simulink model "Copy_of_PDUSTM32"  (R2024b)
settings: Solver=FixedStepDiscrete  StartTime=0.0  StopTime=1  FixedStep=0.001  RelTol=1e-3  EnableMultiTasking=on
libraries: stm32blockslib x32, stm32f4xxblockslib x14, canmsglib x7, simulink x3, stm32h7xxblockslib x1
(part 2 of 3)

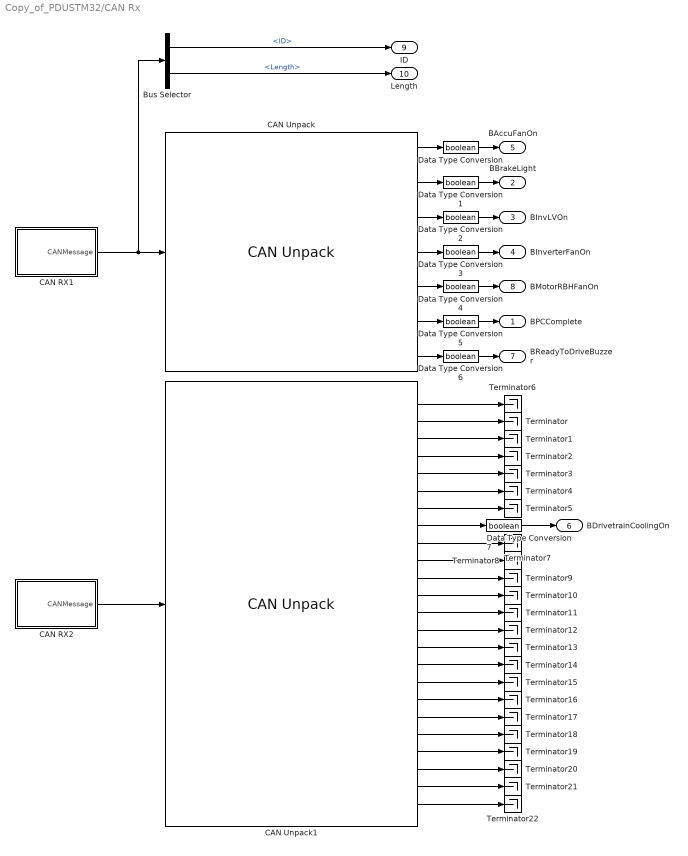
== system Copy_of_PDUSTM32/CAN Rx ==
  Bus Selector : BusSelector  OutputSignals=ID,Length
  CAN RX1 : Subsystem  mask{SPIModuleSelect=SPI1, Port_Select=GPIOB, Pin=14, PortName=GPIOB, PinNumber=2}
      mask prompts: SPIModuleSelect "SPI Module"; Port_Select "CS Port"; Pin "CS Pin"; PortName "INT Port"; PinNumber "INT Pin"
      mask TypeOptions SPIModuleSelect:
      | Enabled
      | Subsystem/SPI Controller Transfer7/SPIModuleSelect
      mask TypeOptions Port_Select:
      | Enabled
      | Subsystem/SPI Controller Transfer7/Port_Select
      mask TypeOptions Pin:
      | Enabled
      | Subsystem/SPI Controller Transfer7/Pin
      mask TypeOptions PortName: Digital Port Read5/PortName
      mask TypeOptions PinNumber: Digital Port Read5/PinNumber
      mask DialogControl DescTextVar Prompt: Read RX buffer when the INT pin is pulled low. Outputs a CANMessage type to be fed into a CAN unpack
      mask Display:
      | %port_label('output', 1, 'CANMessage');
      | 
      | text(0.05, 0.5, '' + string(get_param(gcb,'SPIModuleSelect')), HorizontalAlignment = 'left');
      | text(0.05, 0.85, 'CS ' + string(get_param(gcb,'Port_Select')) + ' Pin ' + string(get_param(gcb,'Pin')), HorizontalAlignment = 'left');
      | 
      | 
      | text(0.05, 0.15, 'INT ' + string(get_param(gcb,'PortName')) + ' Pin ' + string(get_param(gcb,'PinNumber')), HorizontalAlignment = 'left');
      | %text(0.05, 0.15, 'INT Pin ' + string(get_param(gcb,'PinNumber')), HorizontalAlignment = 'left');
      | 
      | 
      | % OBR logo
      | pos = get_param(gcb, 'Position');
      | blockAspect = (pos(3)-pos(1)) / (pos(4)-pos(2));
      | 
      | % fit(img, m, cx, cy): m = fraction of block the image occupies,
      | % (cx,cy) = center point in normalized 0-1 coords
      | fit = @(img,m,cx,cy) [ ...
      |     cx - m*min(1,(size(img,2)/size(img,1))/blockAspect)/2, ...
      |     cy - m*min(1,blockAspect/(size(img,2)/size(img,1)))/2, ...
      |     m*min(1,(size(img,2)/size(img,1))/blockAspect), ...
      |     m*min(1,blockAspect/(size(img,2)/size(img,1))) ];
      | 
      | ud = get_param(gcb, 'UserData');
      | 
      | image(ud.mcplogo, fit(ud.mcplogo, 0.3, 0.85, 0.5));
      | image(ud.obrlogo, fit(ud.obrlogo, 0.5, 0.5, 0.5));
  CAN RX2 : Subsystem  mask{SPIModuleSelect=SPI1, Port_Select=GPIOB, Pin=14, PortName=GPIOB, PinNumber=2}
      mask prompts: SPIModuleSelect "SPI Module"; Port_Select "CS Port"; Pin "CS Pin"; PortName "INT Port"; PinNumber "INT Pin"
      mask TypeOptions SPIModuleSelect:
      | Enabled
      | Subsystem/SPI Controller Transfer7/SPIModuleSelect
      mask TypeOptions Port_Select:
      | Enabled
      | Subsystem/SPI Controller Transfer7/Port_Select
      mask TypeOptions Pin:
      | Enabled
      | Subsystem/SPI Controller Transfer7/Pin
      mask TypeOptions PortName: Digital Port Read5/PortName
      mask TypeOptions PinNumber: Digital Port Read5/PinNumber
      mask DialogControl DescTextVar Prompt: Read RX buffer when the INT pin is pulled low. Outputs a CANMessage type to be fed into a CAN unpack
      mask Display:
      | %port_label('output', 1, 'CANMessage');
      | 
      | text(0.05, 0.5, '' + string(get_param(gcb,'SPIModuleSelect')), HorizontalAlignment = 'left');
      | text(0.05, 0.85, 'CS ' + string(get_param(gcb,'Port_Select')) + ' Pin ' + string(get_param(gcb,'Pin')), HorizontalAlignment = 'left');
      | 
      | 
      | text(0.05, 0.15, 'INT ' + string(get_param(gcb,'PortName')) + ' Pin ' + string(get_param(gcb,'PinNumber')), HorizontalAlignment = 'left');
      | %text(0.05, 0.15, 'INT Pin ' + string(get_param(gcb,'PinNumber')), HorizontalAlignment = 'left');
      | 
      | 
      | % OBR logo
      | pos = get_param(gcb, 'Position');
      | blockAspect = (pos(3)-pos(1)) / (pos(4)-pos(2));
      | 
      | % fit(img, m, cx, cy): m = fraction of block the image occupies,
      | % (cx,cy) = center point in normalized 0-1 coords
      | fit = @(img,m,cx,cy) [ ...
      |     cx - m*min(1,(size(img,2)/size(img,1))/blockAspect)/2, ...
      |     cy - m*min(1,blockAspect/(size(img,2)/size(img,1)))/2, ...
      |     m*min(1,(size(img,2)/size(img,1))/blockAspect), ...
      |     m*min(1,blockAspect/(size(img,2)/size(img,1))) ];
      | 
      | ud = get_param(gcb, 'UserData');
      | 
      | image(ud.mcplogo, fit(ud.mcplogo, 0.3, 0.85, 0.5));
      | image(ud.obrlogo, fit(ud.obrlogo, 0.5, 0.5, 0.5));
  CAN Unpack : canmsglib/CAN Unpack  CANdbFile=C:\Users\oxbro\Documents\STM32CustomProjects\PDUSTM32\CAN3_28.06.26.dbc  MsgList=VCU_PDMReq  MsgName=VCU_PDMReq  MsgIDType=Standard (11-bit identifier)  MsgIdentifier=1539  MsgLength=7  SignalInfo={'BAccuFanOn','24','1','LE','unsigned','Standard','0','1','0','0','1';'BBrakeLight','0','1','LE','unsigned','Standard','0','1','0','0','1';'BInvLVOn','32','1','LE','unsigned','Standard','0','1','0','0','1';'BInverterFanOn','8','1','LE','unsigned','Standard','0','1','0','0','1';'BMotorRBHFanOn','16','1','LE','unsigned','Standard','0','1','0','0','1';'BPCComplete','40','1','LE','unsigned','Standard','0','1','0','0','1';'BReadyToDriveBuzzer','48','1','LE','unsigned','Standard','0','1','0','0','1'}  IDPort=off  TimestampPort=off  ErrorPort=off  RemotePort=off  LengthPort=off  StatusPort=off  ApplyMinMax=off
      settings: LibrarySourceBlock=stmutilitieslib/CAN Unpack  DataFormat=CANdb specified signals
  CAN Unpack1 : canmsglib/CAN Unpack  CANdbFile=C:\Users\will\Desktop\STM32Projects\PDUSTM32\CAN3_28.06.26.dbc  MsgList=VCU_1s_Frame4  MsgName=VCU_1s_Frame4  MsgIDType=Standard (11-bit identifier)  MsgIdentifier=419  MsgLength=6  SignalInfo={'BBMSP0A0COut','32','1','LE','unsigned','Standard','0','1','0','0','1';'BBMSP0A0EOut','33','1','LE','unsigned','Standard','0','1','0','0','1';'BBMSP0A10Out','34','1','LE','unsigned','Standard','0','1','0','0','1';'BBMSP0A80Out','35','1','LE','unsigned','Standard','0','1','0','0','1';'BBMSP0AC0Out','36','1','LE','unsigned','Standard','0','1','0','0','1';'BBMSP0AFAOut','37','1','LE','unsigned','Standard','0','1','0','0','1';'BBalancingOnOut','31','1','LE','unsigned','Standard','0','1','0','0','1';'BDrivetrainCoolingOn','1','1','LE','unsigned','Standard','0','1','0','0','1';'BDrivetrainCoolingOnEM','5','1','LE','unsigned','Standard','0','1','0','0','1';'BDrivetrainCoolingOnOW','6','2','LE','unsigned','Standard','0','1','-1','-1','2';'BEMSOn','13','1','LE','unsigned','Standard','0','1','0','0','1';'BEMSOnEM','14','1','LE','unsigned','Standard','0','1','0','0','1';'BEMSOnOW','15','2','LE','unsigned','Standard','0','1','-1','-1','2';'BSpinningModeOn','17','1','LE','unsigned','Standard','0','1','0','0','1';'BSpinningModeOnEM','18','1','LE','unsigned','Standard','0','1','0','0','1';'BSpinningModeOnOW','19','2','LE','unsigned','Standard','0','1','-1','-1','2';'BTCOn','9','1','LE','unsigned','Standard','0','1','0','0','1';'BTCOnEM','10','1','LE','unsigned','Standard','0','1','0','0','1';'BTCOnOW','11','2','LE','unsigned','Standard','0','1','-1','-1','2';'BTVOnEM','0','1','LE','unsigned','Standard','0','1','0','0','1';'BTVOnOW','2','2','LE','unsigned','Standard','0','1','-1','-1','2';'NEventMode','44','4','LE','unsigned','Standard','0','1','0','0','15';'NLap','38','6','LE','unsigned','Standard','0','1','0','0','63';'rSoE','21','10','LE','unsigned','Standard','0','0.1','0','0','102.3'}  IDPort=off  TimestampPort=off  ErrorPort=off  RemotePort=off  LengthPort=off  StatusPort=off  ApplyMinMax=off
      settings: LibrarySourceBlock=stmutilitieslib/CAN Unpack  DataFormat=CANdb specified signals
  Data Type Conversion{,1..7} (8 alike) : DataTypeConversion  OutDataTypeStr=boolean  SaturateOnIntegerOverflow=off  RndMeth=Floor
  Terminator{,1..22} (23 alike) : Terminator
  BPCComplete : Outport  OutDataTypeStr=boolean
  BBrakeLight : Outport  Port=2  OutDataTypeStr=boolean
  BInvLVOn : Outport  Port=3  OutDataTypeStr=boolean
  BInverterFanOn : Outport  Port=4  OutDataTypeStr=boolean
  BAccuFanOn : Outport  Port=5  OutDataTypeStr=boolean
  BDrivetrainCoolingOn : Outport  Port=6  OutDataTypeStr=boolean
  BReadyToDriveBuzzer : Outport  Port=7  OutDataTypeStr=boolean
  BMotorRBHFanOn : Outport  Port=8  OutDataTypeStr=boolean
  ID : Outport  Port=9
  Length : Outport  Port=10
  wires:
  CAN RX1/1(CANMessage) -> Bus Selector/1, CAN Unpack/1
  CAN Unpack/1 -> Data Type Conversion/1
  CAN Unpack/2 -> Data Type Conversion1/1
  CAN Unpack1/2 -> Terminator/1
  CAN Unpack1/3 -> Terminator1/1
  CAN Unpack1/4 -> Terminator2/1
  CAN Unpack1/5 -> Terminator3/1
  CAN Unpack1/6 -> Terminator4/1
  CAN Unpack1/7 -> Terminator5/1
  CAN Unpack1/9 -> Terminator7/1
  CAN Unpack1/10 -> Terminator8/1
  CAN Unpack1/19 -> Terminator17/1
  CAN Unpack1/18 -> Terminator16/1
  CAN Unpack1/17 -> Terminator15/1
  CAN Unpack1/16 -> Terminator14/1
  CAN Unpack1/15 -> Terminator13/1
  CAN Unpack1/14 -> Terminator12/1
  CAN Unpack1/13 -> Terminator11/1
  CAN Unpack1/12 -> Terminator10/1
  CAN Unpack1/20 -> Terminator18/1
  CAN Unpack1/21 -> Terminator19/1
  CAN Unpack1/22 -> Terminator20/1
  CAN Unpack1/23 -> Terminator21/1
  CAN Unpack1/24 -> Terminator22/1
  CAN Unpack1/11 -> Terminator9/1
  CAN Unpack1/1 -> Terminator6/1
  Data Type Conversion/1 -> BAccuFanOn/1
  Data Type Conversion1/1 -> BBrakeLight/1
  Data Type Conversion2/1 -> BInvLVOn/1
  Data Type Conversion3/1 -> BInverterFanOn/1
  Data Type Conversion4/1 -> BMotorRBHFanOn/1
  Data Type Conversion6/1 -> BReadyToDriveBuzzer/1
  Data Type Conversion7/1 -> BDrivetrainCoolingOn/1
  Data Type Conversion5/1 -> BPCComplete/1
  CAN Unpack1/8 -> Data Type Conversion7/1
  CAN Unpack/7 -> Data Type Conversion6/1
  Bus Selector/1 -> ID/1  "<ID>"
  Bus Selector/2 -> Length/1  "<Length>"
  CAN RX2/1(CANMessage) -> CAN Unpack1/1
  CAN Unpack/3 -> Data Type Conversion2/1
  CAN Unpack/4 -> Data Type Conversion3/1
  CAN Unpack/5 -> Data Type Conversion4/1
  CAN Unpack/6 -> Data Type Conversion5/1

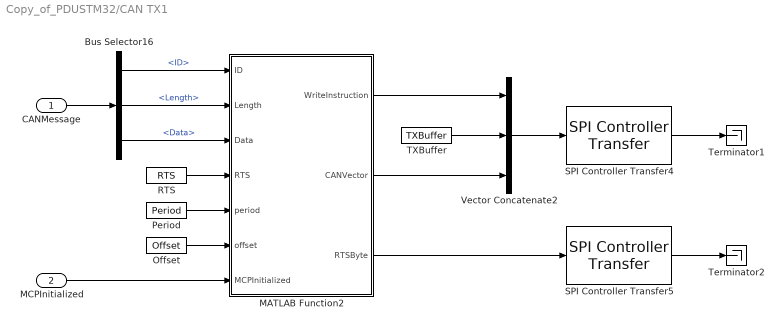
== system Copy_of_PDUSTM32/CAN TX1 ==
  CANMessage : Inport
  MCPInitialized : Inport  Port=2
  Bus Selector16 : BusSelector  OutputSignals=ID,Length,Data
  MATLAB Function2 : MATLAB Function  TreatAsAtomicUnit=on
  Offset : Constant  Value=Offset  OutDataTypeStr=uint16  SampleTime=-1
  Period : Constant  Value=Period  OutDataTypeStr=uint16  SampleTime=-1
  RTS : Constant  Value=RTS  OutDataTypeStr=uint8  SampleTime=-1
  SPI Controller Transfer4 : stm32blockslib/SPI Controller Transfer  Priority=1  SPIModuleSelect=SPI1  ClockPolarity=Low  ClockPhase=1 Edge  SPIModule=SPIModule  Mode=Master  BusSpeed=uint32(1000000)  FirstBitToTransfer=Most significant bit (MSB)  ClockMode=0  BlockFunction=Transfer  EnableRegisterAddress=off  RegisterAddress=0  OutputDataType=uint8  OutputDataLength=1  OutputStatus=off  BlockingMode=off  Timeout=0.01  DataBits=8  UseCustomSSPin=Explicit GPIO calls  ActiveLowSSPin=Active low  Port_Select=GPIOB  Pin=Pin
      settings: LibrarySourceBlock=stm32h7xxblockslib/SPI Controller Transfer
  SPI Controller Transfer5 : stm32blockslib/SPI Controller Transfer  Priority=2  SPIModuleSelect=SPI1  ClockPolarity=Low  ClockPhase=1 Edge  SPIModule=SPIModule  Mode=Master  BusSpeed=uint32(1000000)  FirstBitToTransfer=Most significant bit (MSB)  ClockMode=0  BlockFunction=Transfer  EnableRegisterAddress=off  RegisterAddress=0  OutputDataType=uint8  OutputDataLength=1  OutputStatus=off  BlockingMode=off  Timeout=0.01  DataBits=8  UseCustomSSPin=Explicit GPIO calls  ActiveLowSSPin=Active low  Port_Select=GPIOB  Pin=Pin
      settings: LibrarySourceBlock=stm32h7xxblockslib/SPI Controller Transfer
  TXBuffer : Constant  Value=TXBuffer  OutDataTypeStr=uint8  SampleTime=-1
  Terminator1 : Terminator
  Terminator2 : Terminator
  Vector Concatenate2 : Concatenate  NumInputs=3
  wires:
  TXBuffer/1 -> Vector Concatenate2/2
  Bus Selector16/1 -> MATLAB Function2/1(ID)  "<ID>"
  RTS/1 -> MATLAB Function2/4(RTS)
  SPI Controller Transfer4/1 -> Terminator1/1
  Vector Concatenate2/1 -> SPI Controller Transfer4/1
  SPI Controller Transfer5/1 -> Terminator2/1
  MATLAB Function2/2(CANVector) -> Vector Concatenate2/3
  MATLAB Function2/1(WriteInstruction) -> Vector Concatenate2/1
  Offset/1 -> MATLAB Function2/6(offset)
  MATLAB Function2/3(RTSByte) -> SPI Controller Transfer5/1
  Period/1 -> MATLAB Function2/5(period)
  Bus Selector16/2 -> MATLAB Function2/2(Length)  "<Length>"
  Bus Selector16/3 -> MATLAB Function2/3(Data)  "<Data>"
  CANMessage/1 -> Bus Selector16/1
  MCPInitialized/1 -> MATLAB Function2/7(MCPInitialized)

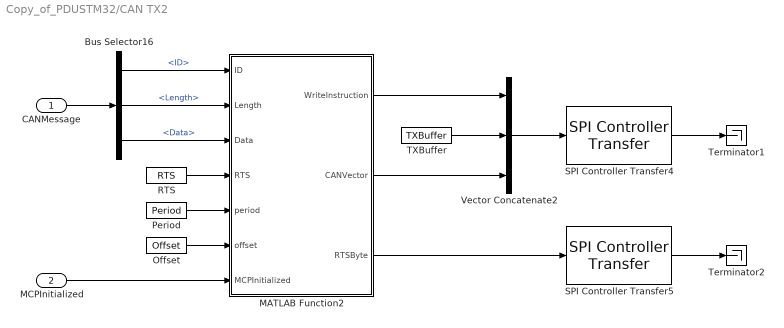
== system Copy_of_PDUSTM32/CAN TX2 ==
  CANMessage : Inport
  MCPInitialized : Inport  Port=2
  Bus Selector16 : BusSelector  OutputSignals=ID,Length,Data
  MATLAB Function2 : MATLAB Function  TreatAsAtomicUnit=on
  Offset : Constant  Value=Offset  OutDataTypeStr=uint16  SampleTime=-1
  Period : Constant  Value=Period  OutDataTypeStr=uint16  SampleTime=-1
  RTS : Constant  Value=RTS  OutDataTypeStr=uint8  SampleTime=-1
  SPI Controller Transfer4 : stm32blockslib/SPI Controller Transfer  Priority=1  SPIModuleSelect=SPI1  ClockPolarity=Low  ClockPhase=1 Edge  SPIModule=SPIModule  Mode=Master  BusSpeed=uint32(1000000)  FirstBitToTransfer=Most significant bit (MSB)  ClockMode=0  BlockFunction=Transfer  EnableRegisterAddress=off  RegisterAddress=0  OutputDataType=uint8  OutputDataLength=1  OutputStatus=off  BlockingMode=off  Timeout=0.01  DataBits=8  UseCustomSSPin=Explicit GPIO calls  ActiveLowSSPin=Active low  Port_Select=GPIOB  Pin=Pin
      settings: LibrarySourceBlock=stm32h7xxblockslib/SPI Controller Transfer
  SPI Controller Transfer5 : stm32blockslib/SPI Controller Transfer  Priority=2  SPIModuleSelect=SPI1  ClockPolarity=Low  ClockPhase=1 Edge  SPIModule=SPIModule  Mode=Master  BusSpeed=uint32(1000000)  FirstBitToTransfer=Most significant bit (MSB)  ClockMode=0  BlockFunction=Transfer  EnableRegisterAddress=off  RegisterAddress=0  OutputDataType=uint8  OutputDataLength=1  OutputStatus=off  BlockingMode=off  Timeout=0.01  DataBits=8  UseCustomSSPin=Explicit GPIO calls  ActiveLowSSPin=Active low  Port_Select=GPIOB  Pin=Pin
      settings: LibrarySourceBlock=stm32h7xxblockslib/SPI Controller Transfer
  TXBuffer : Constant  Value=TXBuffer  OutDataTypeStr=uint8  SampleTime=-1
  Terminator1 : Terminator
  Terminator2 : Terminator
  Vector Concatenate2 : Concatenate  NumInputs=3
  wires:
  TXBuffer/1 -> Vector Concatenate2/2
  Bus Selector16/1 -> MATLAB Function2/1(ID)  "<ID>"
  RTS/1 -> MATLAB Function2/4(RTS)
  SPI Controller Transfer4/1 -> Terminator1/1
  Vector Concatenate2/1 -> SPI Controller Transfer4/1
  SPI Controller Transfer5/1 -> Terminator2/1
  MATLAB Function2/2(CANVector) -> Vector Concatenate2/3
  MATLAB Function2/1(WriteInstruction) -> Vector Concatenate2/1
  Offset/1 -> MATLAB Function2/6(offset)
  MATLAB Function2/3(RTSByte) -> SPI Controller Transfer5/1
  Period/1 -> MATLAB Function2/5(period)
  Bus Selector16/2 -> MATLAB Function2/2(Length)  "<Length>"
  Bus Selector16/3 -> MATLAB Function2/3(Data)  "<Data>"
  CANMessage/1 -> Bus Selector16/1
  MCPInitialized/1 -> MATLAB Function2/7(MCPInitialized)

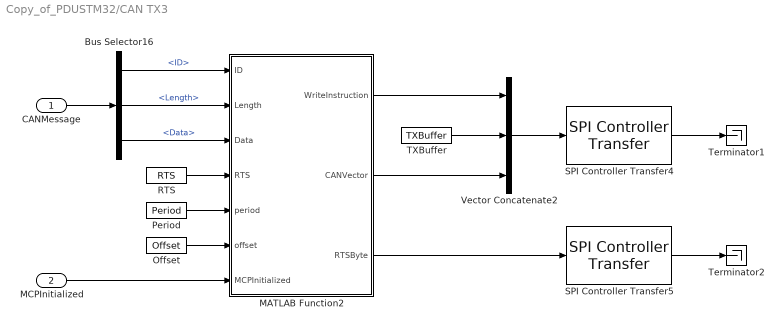
== system Copy_of_PDUSTM32/CAN TX3 ==
  CANMessage : Inport
  MCPInitialized : Inport  Port=2
  Bus Selector16 : BusSelector  OutputSignals=ID,Length,Data
  MATLAB Function2 : MATLAB Function  TreatAsAtomicUnit=on
  Offset : Constant  Value=Offset  OutDataTypeStr=uint16  SampleTime=-1
  Period : Constant  Value=Period  OutDataTypeStr=uint16  SampleTime=-1
  RTS : Constant  Value=RTS  OutDataTypeStr=uint8  SampleTime=-1
  SPI Controller Transfer4 : stm32blockslib/SPI Controller Transfer  Priority=1  SPIModuleSelect=SPI1  ClockPolarity=Low  ClockPhase=1 Edge  SPIModule=SPIModule  Mode=Master  BusSpeed=uint32(1000000)  FirstBitToTransfer=Most significant bit (MSB)  ClockMode=0  BlockFunction=Transfer  EnableRegisterAddress=off  RegisterAddress=0  OutputDataType=uint8  OutputDataLength=1  OutputStatus=off  BlockingMode=off  Timeout=0.01  DataBits=8  UseCustomSSPin=Explicit GPIO calls  ActiveLowSSPin=Active low  Port_Select=GPIOB  Pin=Pin
      settings: LibrarySourceBlock=stm32h7xxblockslib/SPI Controller Transfer
  SPI Controller Transfer5 : stm32blockslib/SPI Controller Transfer  Priority=2  SPIModuleSelect=SPI1  ClockPolarity=Low  ClockPhase=1 Edge  SPIModule=SPIModule  Mode=Master  BusSpeed=uint32(1000000)  FirstBitToTransfer=Most significant bit (MSB)  ClockMode=0  BlockFunction=Transfer  EnableRegisterAddress=off  RegisterAddress=0  OutputDataType=uint8  OutputDataLength=1  OutputStatus=off  BlockingMode=off  Timeout=0.01  DataBits=8  UseCustomSSPin=Explicit GPIO calls  ActiveLowSSPin=Active low  Port_Select=GPIOB  Pin=Pin
      settings: LibrarySourceBlock=stm32h7xxblockslib/SPI Controller Transfer
  TXBuffer : Constant  Value=TXBuffer  OutDataTypeStr=uint8  SampleTime=-1
  Terminator1 : Terminator
  Terminator2 : Terminator
  Vector Concatenate2 : Concatenate  NumInputs=3
  wires:
  TXBuffer/1 -> Vector Concatenate2/2
  Bus Selector16/1 -> MATLAB Function2/1(ID)  "<ID>"
  RTS/1 -> MATLAB Function2/4(RTS)
  SPI Controller Transfer4/1 -> Terminator1/1
  Vector Concatenate2/1 -> SPI Controller Transfer4/1
  SPI Controller Transfer5/1 -> Terminator2/1
  MATLAB Function2/2(CANVector) -> Vector Concatenate2/3
  MATLAB Function2/1(WriteInstruction) -> Vector Concatenate2/1
  Offset/1 -> MATLAB Function2/6(offset)
  MATLAB Function2/3(RTSByte) -> SPI Controller Transfer5/1
  Period/1 -> MATLAB Function2/5(period)
  Bus Selector16/2 -> MATLAB Function2/2(Length)  "<Length>"
  Bus Selector16/3 -> MATLAB Function2/3(Data)  "<Data>"
  CANMessage/1 -> Bus Selector16/1
  MCPInitialized/1 -> MATLAB Function2/7(MCPInitialized)

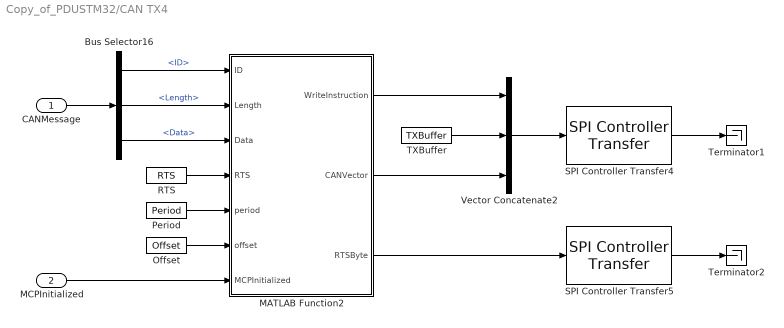
== system Copy_of_PDUSTM32/CAN TX4 ==
  CANMessage : Inport
  MCPInitialized : Inport  Port=2
  Bus Selector16 : BusSelector  OutputSignals=ID,Length,Data
  MATLAB Function2 : MATLAB Function  TreatAsAtomicUnit=on
  Offset : Constant  Value=Offset  OutDataTypeStr=uint16  SampleTime=-1
  Period : Constant  Value=Period  OutDataTypeStr=uint16  SampleTime=-1
  RTS : Constant  Value=RTS  OutDataTypeStr=uint8  SampleTime=-1
  SPI Controller Transfer4 : stm32blockslib/SPI Controller Transfer  Priority=1  SPIModuleSelect=SPI1  ClockPolarity=Low  ClockPhase=1 Edge  SPIModule=SPIModule  Mode=Master  BusSpeed=uint32(1000000)  FirstBitToTransfer=Most significant bit (MSB)  ClockMode=0  BlockFunction=Transfer  EnableRegisterAddress=off  RegisterAddress=0  OutputDataType=uint8  OutputDataLength=1  OutputStatus=off  BlockingMode=off  Timeout=0.01  DataBits=8  UseCustomSSPin=Explicit GPIO calls  ActiveLowSSPin=Active low  Port_Select=GPIOB  Pin=Pin
      settings: LibrarySourceBlock=stm32h7xxblockslib/SPI Controller Transfer
  SPI Controller Transfer5 : stm32blockslib/SPI Controller Transfer  Priority=2  SPIModuleSelect=SPI1  ClockPolarity=Low  ClockPhase=1 Edge  SPIModule=SPIModule  Mode=Master  BusSpeed=uint32(1000000)  FirstBitToTransfer=Most significant bit (MSB)  ClockMode=0  BlockFunction=Transfer  EnableRegisterAddress=off  RegisterAddress=0  OutputDataType=uint8  OutputDataLength=1  OutputStatus=off  BlockingMode=off  Timeout=0.01  DataBits=8  UseCustomSSPin=Explicit GPIO calls  ActiveLowSSPin=Active low  Port_Select=GPIOB  Pin=Pin
      settings: LibrarySourceBlock=stm32h7xxblockslib/SPI Controller Transfer
  TXBuffer : Constant  Value=TXBuffer  OutDataTypeStr=uint8  SampleTime=-1
  Terminator1 : Terminator
  Terminator2 : Terminator
  Vector Concatenate2 : Concatenate  NumInputs=3
  wires:
  TXBuffer/1 -> Vector Concatenate2/2
  Bus Selector16/1 -> MATLAB Function2/1(ID)  "<ID>"
  RTS/1 -> MATLAB Function2/4(RTS)
  SPI Controller Transfer4/1 -> Terminator1/1
  Vector Concatenate2/1 -> SPI Controller Transfer4/1
  SPI Controller Transfer5/1 -> Terminator2/1
  MATLAB Function2/2(CANVector) -> Vector Concatenate2/3
  MATLAB Function2/1(WriteInstruction) -> Vector Concatenate2/1
  Offset/1 -> MATLAB Function2/6(offset)
  MATLAB Function2/3(RTSByte) -> SPI Controller Transfer5/1
  Period/1 -> MATLAB Function2/5(period)
  Bus Selector16/2 -> MATLAB Function2/2(Length)  "<Length>"
  Bus Selector16/3 -> MATLAB Function2/3(Data)  "<Data>"
  CANMessage/1 -> Bus Selector16/1
  MCPInitialized/1 -> MATLAB Function2/7(MCPInitialized)

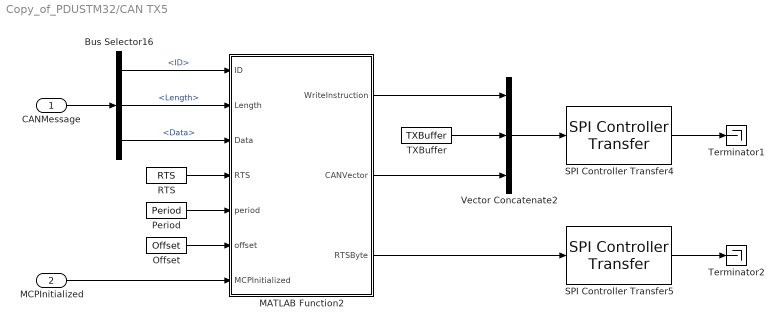
== system Copy_of_PDUSTM32/CAN TX5 ==
  CANMessage : Inport
  MCPInitialized : Inport  Port=2
  Bus Selector16 : BusSelector  OutputSignals=ID,Length,Data
  MATLAB Function2 : MATLAB Function  TreatAsAtomicUnit=on
  Offset : Constant  Value=Offset  OutDataTypeStr=uint16  SampleTime=-1
  Period : Constant  Value=Period  OutDataTypeStr=uint16  SampleTime=-1
  RTS : Constant  Value=RTS  OutDataTypeStr=uint8  SampleTime=-1
  SPI Controller Transfer4 : stm32blockslib/SPI Controller Transfer  Priority=1  SPIModuleSelect=SPI1  ClockPolarity=Low  ClockPhase=1 Edge  SPIModule=SPIModule  Mode=Master  BusSpeed=uint32(1000000)  FirstBitToTransfer=Most significant bit (MSB)  ClockMode=0  BlockFunction=Transfer  EnableRegisterAddress=off  RegisterAddress=0  OutputDataType=uint8  OutputDataLength=1  OutputStatus=off  BlockingMode=off  Timeout=0.01  DataBits=8  UseCustomSSPin=Explicit GPIO calls  ActiveLowSSPin=Active low  Port_Select=GPIOB  Pin=Pin
      settings: LibrarySourceBlock=stm32h7xxblockslib/SPI Controller Transfer
  SPI Controller Transfer5 : stm32blockslib/SPI Controller Transfer  Priority=2  SPIModuleSelect=SPI1  ClockPolarity=Low  ClockPhase=1 Edge  SPIModule=SPIModule  Mode=Master  BusSpeed=uint32(1000000)  FirstBitToTransfer=Most significant bit (MSB)  ClockMode=0  BlockFunction=Transfer  EnableRegisterAddress=off  RegisterAddress=0  OutputDataType=uint8  OutputDataLength=1  OutputStatus=off  BlockingMode=off  Timeout=0.01  DataBits=8  UseCustomSSPin=Explicit GPIO calls  ActiveLowSSPin=Active low  Port_Select=GPIOB  Pin=Pin
      settings: LibrarySourceBlock=stm32h7xxblockslib/SPI Controller Transfer
  TXBuffer : Constant  Value=TXBuffer  OutDataTypeStr=uint8  SampleTime=-1
  Terminator1 : Terminator
  Terminator2 : Terminator
  Vector Concatenate2 : Concatenate  NumInputs=3
  wires:
  TXBuffer/1 -> Vector Concatenate2/2
  Bus Selector16/1 -> MATLAB Function2/1(ID)  "<ID>"
  RTS/1 -> MATLAB Function2/4(RTS)
  SPI Controller Transfer4/1 -> Terminator1/1
  Vector Concatenate2/1 -> SPI Controller Transfer4/1
  SPI Controller Transfer5/1 -> Terminator2/1
  MATLAB Function2/2(CANVector) -> Vector Concatenate2/3
  MATLAB Function2/1(WriteInstruction) -> Vector Concatenate2/1
  Offset/1 -> MATLAB Function2/6(offset)
  MATLAB Function2/3(RTSByte) -> SPI Controller Transfer5/1
  Period/1 -> MATLAB Function2/5(period)
  Bus Selector16/2 -> MATLAB Function2/2(Length)  "<Length>"
  Bus Selector16/3 -> MATLAB Function2/3(Data)  "<Data>"
  CANMessage/1 -> Bus Selector16/1
  MCPInitialized/1 -> MATLAB Function2/7(MCPInitialized)

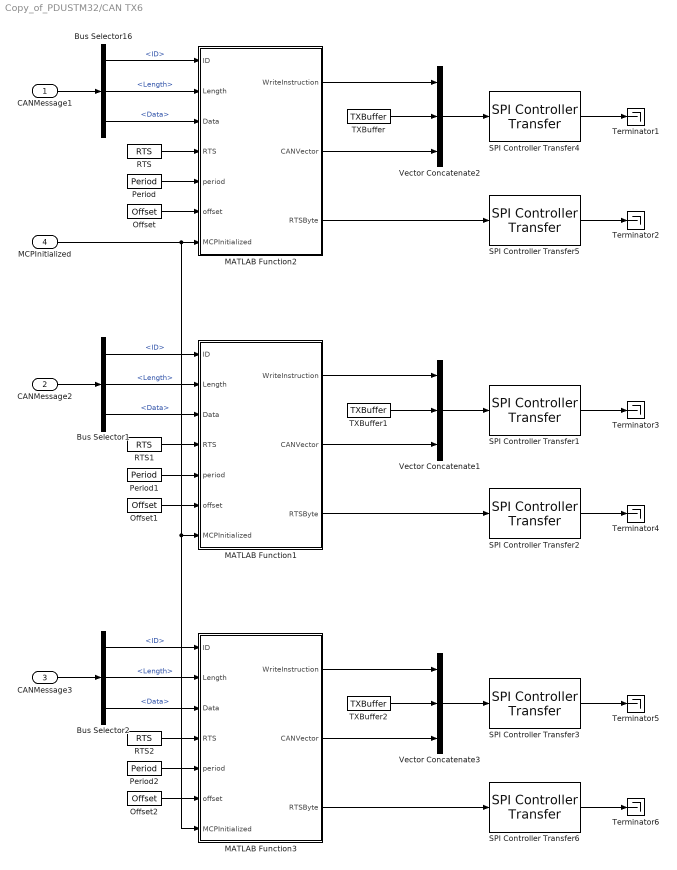
== system Copy_of_PDUSTM32/CAN TX6 ==
  CANMessage1 : Inport
  CANMessage2 : Inport  Port=2
  CANMessage3 : Inport  Port=3
  MCPInitialized : Inport  Port=4
  Bus Selector1 : BusSelector  OutputSignals=ID,Length,Data
  Bus Selector16 : BusSelector  OutputSignals=ID,Length,Data
  Bus Selector2 : BusSelector  OutputSignals=ID,Length,Data
  MATLAB Function1 : MATLAB Function  TreatAsAtomicUnit=on
  MATLAB Function2 : MATLAB Function  TreatAsAtomicUnit=on
  MATLAB Function3 : MATLAB Function  TreatAsAtomicUnit=on
  Offset : Constant  Value=Offset  OutDataTypeStr=uint16  SampleTime=-1
  Offset1 : Constant  Value=Offset  OutDataTypeStr=uint16  SampleTime=-1
  Offset2 : Constant  Value=Offset  OutDataTypeStr=uint16  SampleTime=-1
  Period : Constant  Value=Period  OutDataTypeStr=uint16  SampleTime=-1
  Period1 : Constant  Value=Period  OutDataTypeStr=uint16  SampleTime=-1
  Period2 : Constant  Value=Period  OutDataTypeStr=uint16  SampleTime=-1
  RTS : Constant  Value=RTS  OutDataTypeStr=uint8  SampleTime=-1
  RTS1 : Constant  Value=RTS  OutDataTypeStr=uint8  SampleTime=-1
  RTS2 : Constant  Value=RTS  OutDataTypeStr=uint8  SampleTime=-1
  SPI Controller Transfer1 : stm32blockslib/SPI Controller Transfer  Priority=3  SPIModuleSelect=SPI1  ClockPolarity=Low  ClockPhase=1 Edge  SPIModule=SPIModule  Mode=Master  BusSpeed=uint32(1000000)  FirstBitToTransfer=Most significant bit (MSB)  ClockMode=0  BlockFunction=Transfer  EnableRegisterAddress=off  RegisterAddress=0  OutputDataType=uint8  OutputDataLength=1  OutputStatus=off  BlockingMode=off  Timeout=0.01  DataBits=8  UseCustomSSPin=Explicit GPIO calls  ActiveLowSSPin=Active low  Port_Select=GPIOB  Pin=Pin
      settings: LibrarySourceBlock=stm32h7xxblockslib/SPI Controller Transfer
  SPI Controller Transfer2 : stm32blockslib/SPI Controller Transfer  Priority=4  SPIModuleSelect=SPI1  ClockPolarity=Low  ClockPhase=1 Edge  SPIModule=SPIModule  Mode=Master  BusSpeed=uint32(1000000)  FirstBitToTransfer=Most significant bit (MSB)  ClockMode=0  BlockFunction=Transfer  EnableRegisterAddress=off  RegisterAddress=0  OutputDataType=uint8  OutputDataLength=1  OutputStatus=off  BlockingMode=off  Timeout=0.01  DataBits=8  UseCustomSSPin=Explicit GPIO calls  ActiveLowSSPin=Active low  Port_Select=GPIOB  Pin=Pin
      settings: LibrarySourceBlock=stm32h7xxblockslib/SPI Controller Transfer
  SPI Controller Transfer3 : stm32blockslib/SPI Controller Transfer  Priority=5  SPIModuleSelect=SPI1  ClockPolarity=Low  ClockPhase=1 Edge  SPIModule=SPIModule  Mode=Master  BusSpeed=uint32(1000000)  FirstBitToTransfer=Most significant bit (MSB)  ClockMode=0  BlockFunction=Transfer  EnableRegisterAddress=off  RegisterAddress=0  OutputDataType=uint8  OutputDataLength=1  OutputStatus=off  BlockingMode=off  Timeout=0.01  DataBits=8  UseCustomSSPin=Explicit GPIO calls  ActiveLowSSPin=Active low  Port_Select=GPIOB  Pin=Pin
      settings: LibrarySourceBlock=stm32h7xxblockslib/SPI Controller Transfer
  SPI Controller Transfer4 : stm32blockslib/SPI Controller Transfer  Priority=1  SPIModuleSelect=SPI1  ClockPolarity=Low  ClockPhase=1 Edge  SPIModule=SPIModule  Mode=Master  BusSpeed=uint32(1000000)  FirstBitToTransfer=Most significant bit (MSB)  ClockMode=0  BlockFunction=Transfer  EnableRegisterAddress=off  RegisterAddress=0  OutputDataType=uint8  OutputDataLength=1  OutputStatus=off  BlockingMode=off  Timeout=0.01  DataBits=8  UseCustomSSPin=Explicit GPIO calls  ActiveLowSSPin=Active low  Port_Select=GPIOB  Pin=Pin
      settings: LibrarySourceBlock=stm32h7xxblockslib/SPI Controller Transfer
  SPI Controller Transfer5 : stm32blockslib/SPI Controller Transfer  Priority=2  SPIModuleSelect=SPI1  ClockPolarity=Low  ClockPhase=1 Edge  SPIModule=SPIModule  Mode=Master  BusSpeed=uint32(1000000)  FirstBitToTransfer=Most significant bit (MSB)  ClockMode=0  BlockFunction=Transfer  EnableRegisterAddress=off  RegisterAddress=0  OutputDataType=uint8  OutputDataLength=1  OutputStatus=off  BlockingMode=off  Timeout=0.01  DataBits=8  UseCustomSSPin=Explicit GPIO calls  ActiveLowSSPin=Active low  Port_Select=GPIOB  Pin=Pin
      settings: LibrarySourceBlock=stm32h7xxblockslib/SPI Controller Transfer
  SPI Controller Transfer6 : stm32blockslib/SPI Controller Transfer  Priority=6  SPIModuleSelect=SPI1  ClockPolarity=Low  ClockPhase=1 Edge  SPIModule=SPIModule  Mode=Master  BusSpeed=uint32(1000000)  FirstBitToTransfer=Most significant bit (MSB)  ClockMode=0  BlockFunction=Transfer  EnableRegisterAddress=off  RegisterAddress=0  OutputDataType=uint8  OutputDataLength=1  OutputStatus=off  BlockingMode=off  Timeout=0.01  DataBits=8  UseCustomSSPin=Explicit GPIO calls  ActiveLowSSPin=Active low  Port_Select=GPIOB  Pin=Pin
      settings: LibrarySourceBlock=stm32h7xxblockslib/SPI Controller Transfer
  TXBuffer : Constant  Value=TXBuffer  OutDataTypeStr=uint8  SampleTime=-1
  TXBuffer1 : Constant  Value=TXBuffer  OutDataTypeStr=uint8  SampleTime=-1
  TXBuffer2 : Constant  Value=TXBuffer  OutDataTypeStr=uint8  SampleTime=-1
  Terminator{1..6} (6 alike) : Terminator
  Vector Concatenate1 : Concatenate  NumInputs=3
  Vector Concatenate2 : Concatenate  NumInputs=3
  Vector Concatenate3 : Concatenate  NumInputs=3
  wires:
  TXBuffer/1 -> Vector Concatenate2/2
  Bus Selector16/1 -> MATLAB Function2/1(ID)  "<ID>"
  RTS/1 -> MATLAB Function2/4(RTS)
  SPI Controller Transfer4/1 -> Terminator1/1
  Vector Concatenate2/1 -> SPI Controller Transfer4/1
  SPI Controller Transfer5/1 -> Terminator2/1
  MATLAB Function2/2(CANVector) -> Vector Concatenate2/3
  MATLAB Function2/1(WriteInstruction) -> Vector Concatenate2/1
  Offset/1 -> MATLAB Function2/6(offset)
  MATLAB Function2/3(RTSByte) -> SPI Controller Transfer5/1
  Period/1 -> MATLAB Function2/5(period)
  Bus Selector16/2 -> MATLAB Function2/2(Length)  "<Length>"
  Bus Selector16/3 -> MATLAB Function2/3(Data)  "<Data>"
  CANMessage1/1 -> Bus Selector16/1
  MCPInitialized/1 -> MATLAB Function3/7(MCPInitialized), MATLAB Function1/7(MCPInitialized), MATLAB Function2/7(MCPInitialized)
  CANMessage2/1 -> Bus Selector1/1
  Period1/1 -> MATLAB Function1/5(period)
  TXBuffer1/1 -> Vector Concatenate1/2
  Bus Selector1/2 -> MATLAB Function1/2(Length)  "<Length>"
  MATLAB Function1/2(CANVector) -> Vector Concatenate1/3
  SPI Controller Transfer2/1 -> Terminator4/1
  RTS1/1 -> MATLAB Function1/4(RTS)
  Bus Selector1/1 -> MATLAB Function1/1(ID)  "<ID>"
  Offset1/1 -> MATLAB Function1/6(offset)
  Vector Concatenate1/1 -> SPI Controller Transfer1/1
  SPI Controller Transfer1/1 -> Terminator3/1
  MATLAB Function1/3(RTSByte) -> SPI Controller Transfer2/1
  Bus Selector1/3 -> MATLAB Function1/3(Data)  "<Data>"
  MATLAB Function1/1(WriteInstruction) -> Vector Concatenate1/1
  CANMessage3/1 -> Bus Selector2/1
  Period2/1 -> MATLAB Function3/5(period)
  TXBuffer2/1 -> Vector Concatenate3/2
  Bus Selector2/2 -> MATLAB Function3/2(Length)  "<Length>"
  MATLAB Function3/2(CANVector) -> Vector Concatenate3/3
  SPI Controller Transfer6/1 -> Terminator6/1
  RTS2/1 -> MATLAB Function3/4(RTS)
  Bus Selector2/1 -> MATLAB Function3/1(ID)  "<ID>"
  Offset2/1 -> MATLAB Function3/6(offset)
  Vector Concatenate3/1 -> SPI Controller Transfer3/1
  SPI Controller Transfer3/1 -> Terminator5/1
  MATLAB Function3/3(RTSByte) -> SPI Controller Transfer6/1
  Bus Selector2/3 -> MATLAB Function3/3(Data)  "<Data>"
  MATLAB Function3/1(WriteInstruction) -> Vector Concatenate3/1

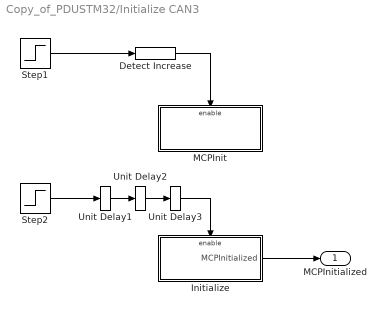
== system Copy_of_PDUSTM32/Initialize CAN3 ==
  Detect Increase : simulink/Logic and Bit Operations/Detect Increase  vinit=0.0  OutDataTypeStr=boolean
  Initialize : Subsystem  TreatAsAtomicUnit=on
  MCPInit : Subsystem  TreatAsAtomicUnit=on
  Step1 : Step
  Step2 : Step
  Unit Delay1 : UnitDelay  SampleTime=-1  HasFrameUpgradeWarning=on
  Unit Delay2 : UnitDelay  SampleTime=-1  HasFrameUpgradeWarning=on
  Unit Delay3 : UnitDelay  SampleTime=-1  HasFrameUpgradeWarning=on
  MCPInitialized : Outport
  wires:
  Detect Increase/1 -> MCPInit/Enable
  Step1/1 -> Detect Increase/1
  Step2/1 -> Unit Delay1/1
  Initialize/1(MCPInitialized) -> MCPInitialized/1
  Unit Delay1/1 -> Unit Delay2/1
  Unit Delay2/1 -> Unit Delay3/1
  Unit Delay3/1 -> Initialize/Enable

== system Copy_of_PDUSTM32/CAN Rx/CAN RX1 ==
  Digital Port Read5 : stm32f4xxblockslib/Digital Port Read  PortName=GPIOB  PinNumber=PinNumber  ReadOperation=on  IOAsArray=off  SampleTime=-1  EnableSimPort=off  hoistedMaskSrc=ECSoC/ECSimCodegen/Digital Port Read
      settings: LibrarySourceBlock=stm32f2xxblockslib/Digital Port Read
  Enabled Subsystem : Subsystem  TreatAsAtomicUnit=on
  NOT5 : Logic  Operator=NOT  IconShape=distinctive  AllPortsSameDT=off  OutDataTypeStr=boolean
  CANMessage : Outport
  wires:
  NOT5/1 -> Enabled Subsystem/Enable
  Digital Port Read5/1 -> NOT5/1
  Enabled Subsystem/1(CANMessage) -> CANMessage/1

== system Copy_of_PDUSTM32/CAN Rx/CAN RX2 ==
  Digital Port Read5 : stm32f4xxblockslib/Digital Port Read  PortName=GPIOB  PinNumber=PinNumber  ReadOperation=on  IOAsArray=off  SampleTime=-1  EnableSimPort=off  hoistedMaskSrc=ECSoC/ECSimCodegen/Digital Port Read
      settings: LibrarySourceBlock=stm32f2xxblockslib/Digital Port Read
  Enabled Subsystem : Subsystem  TreatAsAtomicUnit=on
  NOT5 : Logic  Operator=NOT  IconShape=distinctive  AllPortsSameDT=off  OutDataTypeStr=boolean
  CANMessage : Outport
  wires:
  NOT5/1 -> Enabled Subsystem/Enable
  Digital Port Read5/1 -> NOT5/1
  Enabled Subsystem/1(CANMessage) -> CANMessage/1

== system Copy_of_PDUSTM32/Initialize CAN3/Initialize ==
  Enable : EnablePort
  Constant : Constant  OutDataTypeStr=boolean
  MCPInitialized : Outport
  wires:
  Constant/1 -> MCPInitialized/1

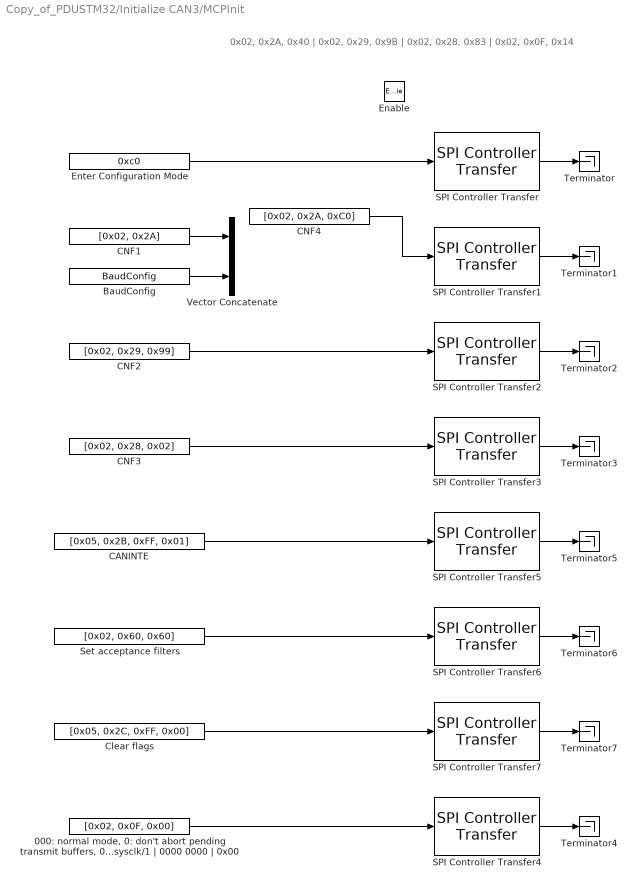
== system Copy_of_PDUSTM32/Initialize CAN3/MCPInit ==
  note: 0x02, 0x2A, 0x40 | 0x02, 0x29, 0x9B | 0x02, 0x28, 0x83 | 0x02, 0x0F, 0x14
  Enable : EnablePort
  " 000: normal mode, 0: don't abort pending transmit buffers, 0: one-shot disabled, 0: CLKOUT disabled, 00: sysclk/1 | 0000 0000 | 0x00" : Constant  Value=[0x02, 0x0F, 0x00]  OutDataTypeStr=uint8
  BaudConfig : Constant  Value=BaudConfig  OutDataTypeStr=uint8
  CANINTE : Constant  Value=[0x05, 0x2B, 0xFF, 0x01]  OutDataTypeStr=uint8
  CNF1 : Constant  Value=[0x02, 0x2A]  OutDataTypeStr=uint8
  CNF2 : Constant  Value=[0x02, 0x29, 0x99]  OutDataTypeStr=uint8
  CNF3 : Constant  Value=[0x02, 0x28, 0x02]  OutDataTypeStr=uint8
  CNF4 : Constant  Value=[0x02, 0x2A, 0xC0]  OutDataTypeStr=uint8
  Clear flags : Constant  Value=[0x05, 0x2C, 0xFF, 0x00]  OutDataTypeStr=uint8
  Enter Configuration Mode : Constant  Value=0xc0  OutDataTypeStr=uint8
  SPI Controller Transfer : stm32blockslib/SPI Controller Transfer  Priority=1  SPIModuleSelect=SPI1  ClockPolarity=Low  ClockPhase=1 Edge  SPIModule=uint32(0)  Mode=Master  BusSpeed=uint32(1000000)  FirstBitToTransfer=Most significant bit (MSB)  ClockMode=0  BlockFunction=Transfer  EnableRegisterAddress=off  RegisterAddress=0  OutputDataType=uint8  OutputDataLength=1  OutputStatus=off  BlockingMode=on  Timeout=0.01  DataBits=8  UseCustomSSPin=Explicit GPIO calls  ActiveLowSSPin=Active low  Port_Select=GPIOB  Pin=Pin
      settings: LibrarySourceBlock=stm32h7xxblockslib/SPI Controller Transfer
  SPI Controller Transfer1 : stm32blockslib/SPI Controller Transfer  Priority=2  SPIModuleSelect=SPI1  ClockPolarity=Low  ClockPhase=1 Edge  SPIModule=uint32(0)  Mode=Master  BusSpeed=uint32(1000000)  FirstBitToTransfer=Most significant bit (MSB)  ClockMode=0  BlockFunction=Transfer  EnableRegisterAddress=off  RegisterAddress=0  OutputDataType=uint8  OutputDataLength=1  OutputStatus=off  BlockingMode=on  Timeout=0.01  DataBits=8  UseCustomSSPin=Explicit GPIO calls  ActiveLowSSPin=Active low  Port_Select=GPIOB  Pin=Pin
      settings: LibrarySourceBlock=stm32h7xxblockslib/SPI Controller Transfer
  SPI Controller Transfer2 : stm32blockslib/SPI Controller Transfer  Priority=3  SPIModuleSelect=SPI1  ClockPolarity=Low  ClockPhase=1 Edge  SPIModule=uint32(0)  Mode=Master  BusSpeed=uint32(1000000)  FirstBitToTransfer=Most significant bit (MSB)  ClockMode=0  BlockFunction=Transfer  EnableRegisterAddress=off  RegisterAddress=0  OutputDataType=uint8  OutputDataLength=1  OutputStatus=off  BlockingMode=on  Timeout=0.01  DataBits=8  UseCustomSSPin=Explicit GPIO calls  ActiveLowSSPin=Active low  Port_Select=GPIOB  Pin=Pin
      settings: LibrarySourceBlock=stm32h7xxblockslib/SPI Controller Transfer
  SPI Controller Transfer3 : stm32blockslib/SPI Controller Transfer  Priority=4  SPIModuleSelect=SPI1  ClockPolarity=Low  ClockPhase=1 Edge  SPIModule=uint32(0)  Mode=Master  BusSpeed=uint32(1000000)  FirstBitToTransfer=Most significant bit (MSB)  ClockMode=0  BlockFunction=Transfer  EnableRegisterAddress=off  RegisterAddress=0  OutputDataType=uint8  OutputDataLength=1  OutputStatus=off  BlockingMode=on  Timeout=0.01  DataBits=8  UseCustomSSPin=Explicit GPIO calls  ActiveLowSSPin=Active low  Port_Select=GPIOB  Pin=Pin
      settings: LibrarySourceBlock=stm32h7xxblockslib/SPI Controller Transfer
  SPI Controller Transfer4 : stm32blockslib/SPI Controller Transfer  Priority=8  SPIModuleSelect=SPI1  ClockPolarity=Low  ClockPhase=1 Edge  SPIModule=uint32(0)  Mode=Master  BusSpeed=uint32(1000000)  FirstBitToTransfer=Most significant bit (MSB)  ClockMode=0  BlockFunction=Transfer  EnableRegisterAddress=off  RegisterAddress=0  OutputDataType=uint8  OutputDataLength=1  OutputStatus=off  BlockingMode=on  Timeout=0.01  DataBits=8  UseCustomSSPin=Explicit GPIO calls  ActiveLowSSPin=Active low  Port_Select=GPIOB  Pin=Pin
      settings: LibrarySourceBlock=stm32h7xxblockslib/SPI Controller Transfer
  SPI Controller Transfer5 : stm32blockslib/SPI Controller Transfer  Priority=5  SPIModuleSelect=SPI1  ClockPolarity=Low  ClockPhase=1 Edge  SPIModule=uint32(0)  Mode=Master  BusSpeed=uint32(1000000)  FirstBitToTransfer=Most significant bit (MSB)  ClockMode=0  BlockFunction=Transfer  EnableRegisterAddress=off  RegisterAddress=0  OutputDataType=uint8  OutputDataLength=1  OutputStatus=off  BlockingMode=on  Timeout=0.01  DataBits=8  UseCustomSSPin=Explicit GPIO calls  ActiveLowSSPin=Active low  Port_Select=GPIOB  Pin=Pin
      settings: LibrarySourceBlock=stm32h7xxblockslib/SPI Controller Transfer
  SPI Controller Transfer6 : stm32blockslib/SPI Controller Transfer  Priority=6  SPIModuleSelect=SPI1  ClockPolarity=Low  ClockPhase=1 Edge  SPIModule=uint32(0)  Mode=Master  BusSpeed=uint32(1000000)  FirstBitToTransfer=Most significant bit (MSB)  ClockMode=0  BlockFunction=Transfer  EnableRegisterAddress=off  RegisterAddress=0  OutputDataType=uint8  OutputDataLength=1  OutputStatus=off  BlockingMode=on  Timeout=0.01  DataBits=8  UseCustomSSPin=Explicit GPIO calls  ActiveLowSSPin=Active low  Port_Select=GPIOB  Pin=Pin
      settings: LibrarySourceBlock=stm32h7xxblockslib/SPI Controller Transfer
  SPI Controller Transfer7 : stm32blockslib/SPI Controller Transfer  Priority=7  SPIModuleSelect=SPI1  ClockPolarity=Low  ClockPhase=1 Edge  SPIModule=uint32(0)  Mode=Master  BusSpeed=uint32(1000000)  FirstBitToTransfer=Most significant bit (MSB)  ClockMode=0  BlockFunction=Transfer  EnableRegisterAddress=off  RegisterAddress=0  OutputDataType=uint8  OutputDataLength=1  OutputStatus=off  BlockingMode=on  Timeout=0.01  DataBits=8  UseCustomSSPin=Explicit GPIO calls  ActiveLowSSPin=Active low  Port_Select=GPIOB  Pin=Pin
      settings: LibrarySourceBlock=stm32h7xxblockslib/SPI Controller Transfer
  Set acceptance filters : Constant  Value=[0x02, 0x60, 0x60]  OutDataTypeStr=uint8
  Terminator{,1..7} (8 alike) : Terminator
  Vector Concatenate : Concatenate
  wires:
  SPI Controller Transfer7/1 -> Terminator7/1
  CNF3/1 -> SPI Controller Transfer3/1
  SPI Controller Transfer6/1 -> Terminator6/1
  CNF2/1 -> SPI Controller Transfer2/1
  CNF4/1 -> SPI Controller Transfer1/1
  SPI Controller Transfer3/1 -> Terminator3/1
  SPI Controller Transfer1/1 -> Terminator1/1
  Clear flags/1 -> SPI Controller Transfer7/1
  SPI Controller Transfer5/1 -> Terminator5/1
  SPI Controller Transfer2/1 -> Terminator2/1
  " 000: normal mode, 0: don't abort pending transmit buffers, 0: one-shot disabled, 0: CLKOUT disabled, 00: sysclk/1 | 0000 0000 | 0x00"/1 -> SPI Controller Transfer4/1
  SPI Controller Transfer4/1 -> Terminator4/1
  CANINTE/1 -> SPI Controller Transfer5/1
  Set acceptance filters/1 -> SPI Controller Transfer6/1
  Enter Configuration Mode/1 -> SPI Controller Transfer/1
  SPI Controller Transfer/1 -> Terminator/1
  BaudConfig/1 -> Vector Concatenate/2
  CNF1/1 -> Vector Concatenate/1

== system Copy_of_PDUSTM32/CAN Rx/CAN RX1/Enabled Subsystem ==
  Enable : EnablePort
  MATLAB Function7 : MATLAB Function  TreatAsAtomicUnit=on
  Read RX Buffer start at RXB0SIDH7 : Constant  Value=uint8([0x90, 0, 0, 0, 0, 0, 0, 0, 0, 0, 0, 0, 0, 0, 0])
  SPI Controller Transfer7 : stm32blockslib/SPI Controller Transfer  Priority=1  SPIModuleSelect=SPI1  ClockPolarity=Low  ClockPhase=1 Edge  SPIModule=uint32(0)  Mode=Master  BusSpeed=uint32(1000000)  FirstBitToTransfer=Most significant bit (MSB)  ClockMode=0  BlockFunction=Transfer  EnableRegisterAddress=off  RegisterAddress=0  OutputDataType=uint8  OutputDataLength=1  OutputStatus=off  BlockingMode=on  Timeout=0.01  DataBits=8  UseCustomSSPin=Explicit GPIO calls  ActiveLowSSPin=Active low  Port_Select=GPIOB  Pin=Pin
      settings: LibrarySourceBlock=stm32h7xxblockslib/SPI Controller Transfer
  CANMessage : Outport
  wires:
  SPI Controller Transfer7/1 -> MATLAB Function7/1(RxBytes)
  Read RX Buffer start at RXB0SIDH7/1 -> SPI Controller Transfer7/1
  MATLAB Function7/1(Message) -> CANMessage/1

== system Copy_of_PDUSTM32/CAN Rx/CAN RX2/Enabled Subsystem ==
  Enable : EnablePort
  MATLAB Function7 : MATLAB Function  TreatAsAtomicUnit=on
  Read RX Buffer start at RXB0SIDH7 : Constant  Value=uint8([0x90, 0, 0, 0, 0, 0, 0, 0, 0, 0, 0, 0, 0, 0, 0])
  SPI Controller Transfer7 : stm32blockslib/SPI Controller Transfer  Priority=1  SPIModuleSelect=SPI1  ClockPolarity=Low  ClockPhase=1 Edge  SPIModule=uint32(0)  Mode=Master  BusSpeed=uint32(1000000)  FirstBitToTransfer=Most significant bit (MSB)  ClockMode=0  BlockFunction=Transfer  EnableRegisterAddress=off  RegisterAddress=0  OutputDataType=uint8  OutputDataLength=1  OutputStatus=off  BlockingMode=on  Timeout=0.01  DataBits=8  UseCustomSSPin=Explicit GPIO calls  ActiveLowSSPin=Active low  Port_Select=GPIOB  Pin=Pin
      settings: LibrarySourceBlock=stm32h7xxblockslib/SPI Controller Transfer
  CANMessage : Outport
  wires:
  SPI Controller Transfer7/1 -> MATLAB Function7/1(RxBytes)
  Read RX Buffer start at RXB0SIDH7/1 -> SPI Controller Transfer7/1
  MATLAB Function7/1(Message) -> CANMessage/1

== matlab function Copy_of_PDUSTM32/CAN TX6/MATLAB Function1 ==
  settings: updateMethod=DISCRETE  sampleTime=.001
  data: WriteInstruction output; ID input uint32; CANVector output uint8; Length input uint8; Data input uint8; RTS input; RTSByte output; period input; offset input; MCPInitialized input
function [WriteInstruction, CANVector, RTSByte] = ConvertToVector(ID, Length, Data, RTS, period, offset, MCPInitialized)
%#codegen
persistent count;
if isempty(count)
    count = uint16(0);
end

if MCPInitialized
    if count == uint16(offset)
        id_u16 = uint16(ID);
        CANVector = zeros(1,13,'uint8');
        CANVector(1) = uint8(bitshift(id_u16, -3));
        CANVector(2) = uint8(bitshift(bitand(id_u16, uint16(7)), 5));
        CANVector(3) = uint8(0);
        CANVector(4) = uint8(0);
        CANVector(5) = bitand(uint8(Length), uint8(15));
        for i = 1:8
            CANVector(5+i) = uint8(Data(i));
        end
        RTSByte = uint8(RTS);
        WriteInstruction = uint8(0x02);
    else
        CANVector = zeros(1,13,'uint8');
        RTSByte = uint8(0x03);
        WriteInstruction = uint8(0x03);
    end

    count = count + uint16(1);
    if count >= uint16(period)
        count = uint16(0);
    end
else
    CANVector = zeros(1,13,'uint8');
    RTSByte = uint8(0x03);
    WriteInstruction = uint8(0x03);
    % don't increment count while MCP not ready
end

== matlab function Copy_of_PDUSTM32/CAN TX6/MATLAB Function3 ==
  settings: updateMethod=DISCRETE  sampleTime=.001
  data: WriteInstruction output; ID input uint32; CANVector output uint8; Length input uint8; Data input uint8; RTS input; RTSByte output; period input; offset input; MCPInitialized input
function [WriteInstruction, CANVector, RTSByte] = ConvertToVector(ID, Length, Data, RTS, period, offset, MCPInitialized)
%#codegen
persistent count;
if isempty(count)
    count = uint16(0);
end

if MCPInitialized
    if count == uint16(offset)
        id_u16 = uint16(ID);
        CANVector = zeros(1,13,'uint8');
        CANVector(1) = uint8(bitshift(id_u16, -3));
        CANVector(2) = uint8(bitshift(bitand(id_u16, uint16(7)), 5));
        CANVector(3) = uint8(0);
        CANVector(4) = uint8(0);
        CANVector(5) = bitand(uint8(Length), uint8(15));
        for i = 1:8
            CANVector(5+i) = uint8(Data(i));
        end
        RTSByte = uint8(RTS);
        WriteInstruction = uint8(0x02);
    else
        CANVector = zeros(1,13,'uint8');
        RTSByte = uint8(0x03);
        WriteInstruction = uint8(0x03);
    end

    count = count + uint16(1);
    if count >= uint16(period)
        count = uint16(0);
    end
else
    CANVector = zeros(1,13,'uint8');
    RTSByte = uint8(0x03);
    WriteInstruction = uint8(0x03);
    % don't increment count while MCP not ready
end

== matlab function Copy_of_PDUSTM32/CAN TX1/MATLAB Function2 ==
  settings: updateMethod=DISCRETE  sampleTime=.001
  data: WriteInstruction output; ID input uint32; CANVector output uint8; Length input uint8; Data input uint8; RTS input; RTSByte output; period input; offset input; MCPInitialized input
function [WriteInstruction, CANVector, RTSByte] = ConvertToVector(ID, Length, Data, RTS, period, offset, MCPInitialized)
%#codegen
persistent count;
if isempty(count)
    count = uint16(0);
end

if MCPInitialized
    if count == uint16(offset)
        id_u16 = uint16(ID);
        CANVector = zeros(1,13,'uint8');
        CANVector(1) = uint8(bitshift(id_u16, -3));
        CANVector(2) = uint8(bitshift(bitand(id_u16, uint16(7)), 5));
        CANVector(3) = uint8(0);
        CANVector(4) = uint8(0);
        CANVector(5) = bitand(uint8(Length), uint8(15));
        for i = 1:8
            CANVector(5+i) = uint8(Data(i));
        end
        RTSByte = uint8(RTS);
        WriteInstruction = uint8(0x02);
    else
        CANVector = zeros(1,13,'uint8');
        RTSByte = uint8(0x03);
        WriteInstruction = uint8(0x03);
    end

    count = count + uint16(1);
    if count >= uint16(period)
        count = uint16(0);
    end
else
    CANVector = zeros(1,13,'uint8');
    RTSByte = uint8(0x03);
    WriteInstruction = uint8(0x03);
    % don't increment count while MCP not ready
end

== matlab function Copy_of_PDUSTM32/CAN Rx/CAN RX1/Enabled Subsystem/MATLAB Function7 ==
  data: RxBytes input uint8 size=15; Message output Bus: CANMessage
function Message = DecodeCANMsg(RxBytes)
%#codegen
% RxBytes is uint8(1x15); bytes 1-2 are don't-care (command echo + one turnaround byte)
SIDH = RxBytes(3);
SIDL = RxBytes(4);
EID8 = RxBytes(5);
EID0 = RxBytes(6);
DLC  = RxBytes(7);

Message.ID       = uint32(bitor(uint32(bitshift(uint32(SIDH), 3)), ...
                        uint32(bitshift(uint32(SIDL), -5))));
Message.Extended = false;
Message.Remote   = false;
Message.Error    = false;
Message.Length   = double(bitand(DLC, uint8(15)));
Message.Data     = RxBytes(8:15);

== matlab function Copy_of_PDUSTM32/CAN TX3/MATLAB Function2 ==
  settings: updateMethod=DISCRETE  sampleTime=.001
  data: WriteInstruction output; ID input uint32; CANVector output uint8; Length input uint8; Data input uint8; RTS input; RTSByte output; period input; offset input; MCPInitialized input
function [WriteInstruction, CANVector, RTSByte] = ConvertToVector(ID, Length, Data, RTS, period, offset, MCPInitialized)
%#codegen
persistent count;
if isempty(count)
    count = uint16(0);
end

if MCPInitialized
    if count == uint16(offset)
        id_u16 = uint16(ID);
        CANVector = zeros(1,13,'uint8');
        CANVector(1) = uint8(bitshift(id_u16, -3));
        CANVector(2) = uint8(bitshift(bitand(id_u16, uint16(7)), 5));
        CANVector(3) = uint8(0);
        CANVector(4) = uint8(0);
        CANVector(5) = bitand(uint8(Length), uint8(15));
        for i = 1:8
            CANVector(5+i) = uint8(Data(i));
        end
        RTSByte = uint8(RTS);
        WriteInstruction = uint8(0x02);
    else
        CANVector = zeros(1,13,'uint8');
        RTSByte = uint8(0x03);
        WriteInstruction = uint8(0x03);
    end

    count = count + uint16(1);
    if count >= uint16(period)
        count = uint16(0);
    end
else
    CANVector = zeros(1,13,'uint8');
    RTSByte = uint8(0x03);
    WriteInstruction = uint8(0x03);
    % don't increment count while MCP not ready
end

== matlab function Copy_of_PDUSTM32/CAN TX4/MATLAB Function2 ==
  settings: updateMethod=DISCRETE  sampleTime=.001
  data: WriteInstruction output; ID input uint32; CANVector output uint8; Length input uint8; Data input uint8; RTS input; RTSByte output; period input; offset input; MCPInitialized input
function [WriteInstruction, CANVector, RTSByte] = ConvertToVector(ID, Length, Data, RTS, period, offset, MCPInitialized)
%#codegen
persistent count;
if isempty(count)
    count = uint16(0);
end

if MCPInitialized
    if count == uint16(offset)
        id_u16 = uint16(ID);
        CANVector = zeros(1,13,'uint8');
        CANVector(1) = uint8(bitshift(id_u16, -3));
        CANVector(2) = uint8(bitshift(bitand(id_u16, uint16(7)), 5));
        CANVector(3) = uint8(0);
        CANVector(4) = uint8(0);
        CANVector(5) = bitand(uint8(Length), uint8(15));
        for i = 1:8
            CANVector(5+i) = uint8(Data(i));
        end
        RTSByte = uint8(RTS);
        WriteInstruction = uint8(0x02);
    else
        CANVector = zeros(1,13,'uint8');
        RTSByte = uint8(0x03);
        WriteInstruction = uint8(0x03);
    end

    count = count + uint16(1);
    if count >= uint16(period)
        count = uint16(0);
    end
else
    CANVector = zeros(1,13,'uint8');
    RTSByte = uint8(0x03);
    WriteInstruction = uint8(0x03);
    % don't increment count while MCP not ready
end
